simulink model "P1"  (R2022b)
settings: Solver=VariableStepAuto  StartTime=0.0  StopTime=10.0  RelTol=1e-3
undefined symbols (not defined in the file): d1, d2, k1, k2, m1, m2
settings Model: Creator=shivavafadar  LastModifiedBy=shivavafadar

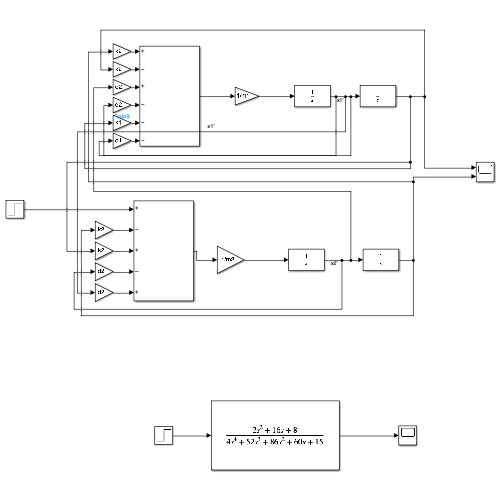
[thumbnail: Simulink's stored preview of the top-level diagram]
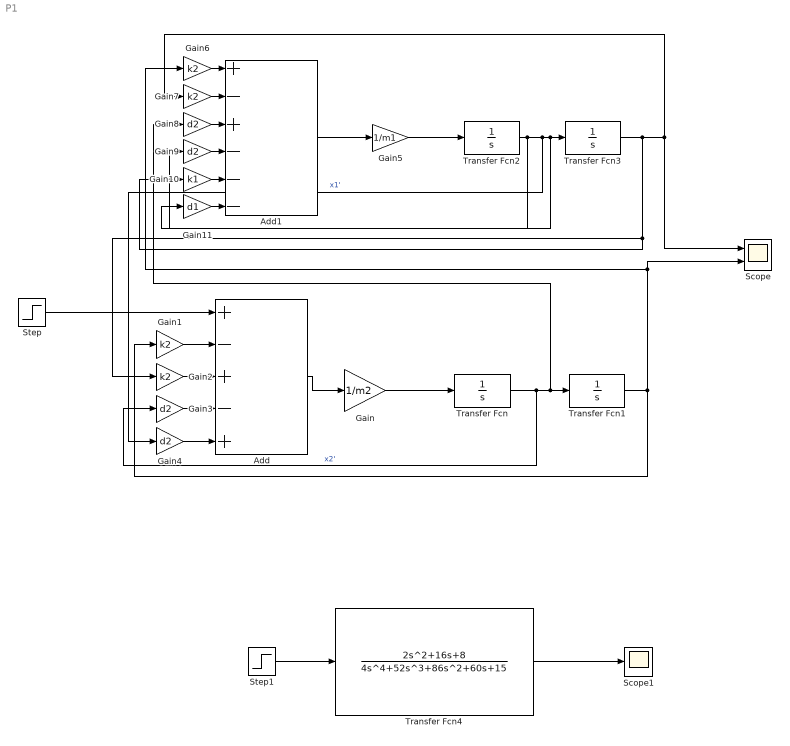
== system P1 ==
  Add : Sum  Inputs=+-+-+
  Add1 : Sum  Inputs=+-+---
  Gain : Gain  Gain=1/m2
  Gain{1..2,6..7} (4 alike) : Gain  Gain=k2
  Gain10 : Gain  Gain=k1
  Gain11 : Gain  Gain=d1
  Gain{3..4,8..9} (4 alike) : Gain  Gain=d2
  Gain5 : Gain  Gain=1/m1
  Scope : Scope  NumInputPorts=2
  Scope1 : Scope
  Step : Step  SampleTime=0
  Step1 : Step  SampleTime=0
  Transfer Fcn{,1..3} (4 alike) : TransferFcn  Denominator=[1 0]
  Transfer Fcn4 : TransferFcn  Numerator=[2 16 8]  Denominator=[4 52 86 60 15]
  wires:
  Transfer Fcn/1 -> Gain3/1, Gain8/1, Transfer Fcn1/1  "x2'"
  Gain/1 -> Transfer Fcn/1
  Transfer Fcn2/1 -> Gain11/1, Gain9/1, Transfer Fcn3/1, Gain4/1  "x1'"
  Gain5/1 -> Transfer Fcn2/1
  Add/1 -> Gain/1
  Step/1 -> Add/1
  Gain1/1 -> Add/2
  Gain2/1 -> Add/3
  Transfer Fcn1/1 -> Scope/2, Gain6/1, Gain1/1
  Transfer Fcn3/1 -> Scope/1, Gain7/1, Gain10/1, Gain2/1
  Gain3/1 -> Add/4
  Gain4/1 -> Add/5
  Add1/1 -> Gain5/1
  Gain6/1 -> Add1/1
  Gain7/1 -> Add1/2
  Gain8/1 -> Add1/3
  Gain9/1 -> Add1/4
  Gain10/1 -> Add1/5
  Gain11/1 -> Add1/6
  Step1/1 -> Transfer Fcn4/1
  Transfer Fcn4/1 -> Scope1/1
